simulink model "simx"  (R2018a)
settings: Solver=VariableStepAuto  StartTime=0.0  StopTime=10  RelTol=1e-3
undefined symbols (not defined in the file): b0, b1, b2
libraries: fuzblock x1
settings Model: Creator=daniel  LastModifiedBy=daniel

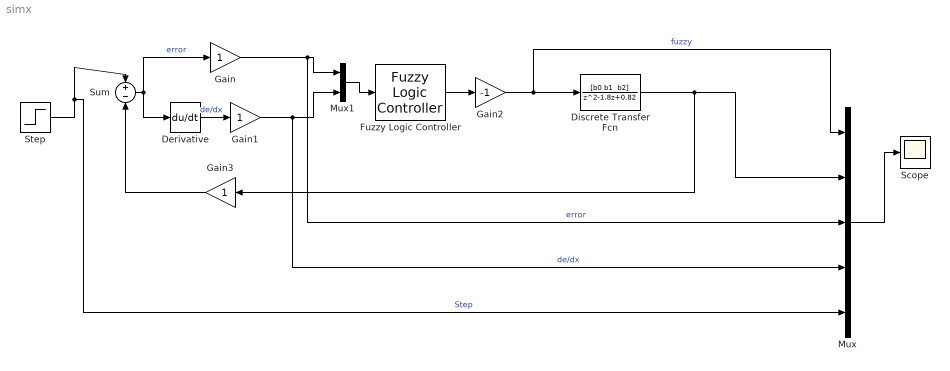
== system simx ==
  Derivative : Derivative
  Discrete Transfer Fcn : DiscreteTransferFcn  Numerator="[b0 b1  b2]"  Denominator=[1 -1.8 0.82]  SampleTime=0.1
  Fuzzy Logic Controller : fuzblock/Fuzzy Logic  Controller  FIS=sys  OutputSampleNumber=101  DataType=double  FuzzifiedInputs=off  RuleFiringStrengths=off  RuleOutputs=off  AggregatedOutputs=off  SimulateUsing=Interpreted execution  OutOfRangeInputValueMessage=warning  NoRuleFiredMessage=warning  EmptyOutputFuzzySetMessage=warning
  Gain : Gain
  Gain1 : Gain
  Gain2 : Gain  Gain=-1
  Gain3 : Gain
  Mux : Mux  Inputs=5
  Mux1 : Mux  Inputs=2
  Scope : Scope
  Step : Step  Time=0  SampleTime=0
  Sum : Sum  Inputs=+-
  wires:
  Mux/1 -> Scope/1
  Step/1 -> Mux/5, Sum/1  "Step"
  Mux1/1 -> Fuzzy Logic Controller/1
  Sum/1 -> Derivative/1, Gain/1  "error"
  Gain1/1 -> Mux/4, Mux1/2  "de/dx"
  Gain/1 -> Mux/3, Mux1/1  "error"
  Gain2/1 -> Discrete Transfer Fcn/1, Mux/1  "fuzzy"
  Fuzzy Logic Controller/1 -> Gain2/1
  Gain3/1 -> Sum/2
  Derivative/1 -> Gain1/1  "de/dx"
  Discrete Transfer Fcn/1 -> Gain3/1, Mux/2
